simulink model "Switching_02"  (R2022b)
settings: Solver=ode4  StartTime=0.0  StopTime=50  FixedStep=1e-3  MaxStep=1e-3  RelTol=1e-3
undefined symbols (not defined in the file or in its folder): p1, p2, p3, PR_kv, PR_kw, SF_b, SF_xi1, v_sat, w_sat, x_d, y_d
libraries: simulink x18, dspsigops x6
settings Model: Creator=david  LastModifiedBy=david

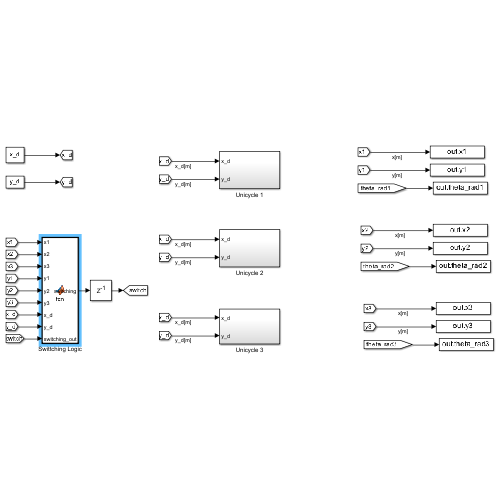
[thumbnail: Simulink's stored preview of the top-level diagram]
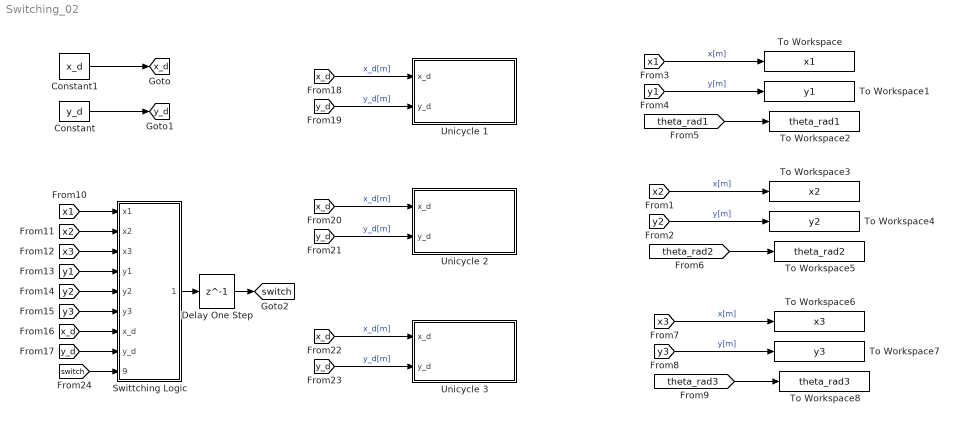
== system Switching_02 ==
  Constant : Constant  Value=y_d
  Constant1 : Constant  Value=x_d
  Delay One Step : Delay  DelayLength=1
  Swittching Logic : MATLAB Function  TreatAsAtomicUnit=on
  To Workspace : ToWorkspace  VariableName=x1  SaveFormat=Structure With Time  SampleTime=-1
  To Workspace1 : ToWorkspace  VariableName=y1  SaveFormat=Structure With Time  SampleTime=-1
  To Workspace2 : ToWorkspace  VariableName=theta_rad1  SaveFormat=Structure With Time  SampleTime=-1
  To Workspace3 : ToWorkspace  VariableName=x2  SaveFormat=Structure With Time  SampleTime=-1
  To Workspace4 : ToWorkspace  VariableName=y2  SaveFormat=Structure With Time  SampleTime=-1
  To Workspace5 : ToWorkspace  VariableName=theta_rad2  SaveFormat=Structure With Time  SampleTime=-1
  To Workspace6 : ToWorkspace  VariableName=x3  SaveFormat=Structure With Time  SampleTime=-1
  To Workspace7 : ToWorkspace  VariableName=y3  SaveFormat=Structure With Time  SampleTime=-1
  To Workspace8 : ToWorkspace  VariableName=theta_rad3  SaveFormat=Structure With Time  SampleTime=-1
  Unicycle 1 : Subsystem
  Unicycle 2 : Subsystem
  Unicycle 3 : Subsystem
  tag scope: switch=global, x_d=global, y_d=global
  wires:
  [x1] -> To Workspace/1  "x[m]"
  [y1] -> To Workspace1/1  "y[m]"
  [theta_rad1] -> To Workspace2/1
  [x2] -> To Workspace3/1  "x[m]"
  [y2] -> To Workspace4/1  "y[m]"
  [theta_rad2] -> To Workspace5/1
  [theta_rad3] -> To Workspace8/1
  [y3] -> To Workspace7/1  "y[m]"
  [x3] -> To Workspace6/1  "x[m]"
  Constant1/1 -> [x_d]
  Constant/1 -> [y_d]
  [x1] -> Swittching Logic/1(x1)
  [x2] -> Swittching Logic/2(x2)
  [x3] -> Swittching Logic/3(x3)
  [y1] -> Swittching Logic/4(y1)
  [y2] -> Swittching Logic/5(y2)
  [y3] -> Swittching Logic/6(y3)
  [x_d] -> Unicycle 1/1(x_d)  "x_d[m]"
  [y_d] -> Unicycle 1/2(y_d)  "y_d[m]"
  [y_d] -> Unicycle 2/2(y_d)  "y_d[m]"
  [x_d] -> Unicycle 2/1(x_d)  "x_d[m]"
  [y_d] -> Unicycle 3/2(y_d)  "y_d[m]"
  [x_d] -> Unicycle 3/1(x_d)  "x_d[m]"
  Swittching Logic/1(switching) -> Delay One Step/1
  [switch] -> Swittching Logic/9(switching_out)
  [y_d] -> Swittching Logic/8(y_d)
  [x_d] -> Swittching Logic/7(x_d)
  Delay One Step/1 -> [switch]

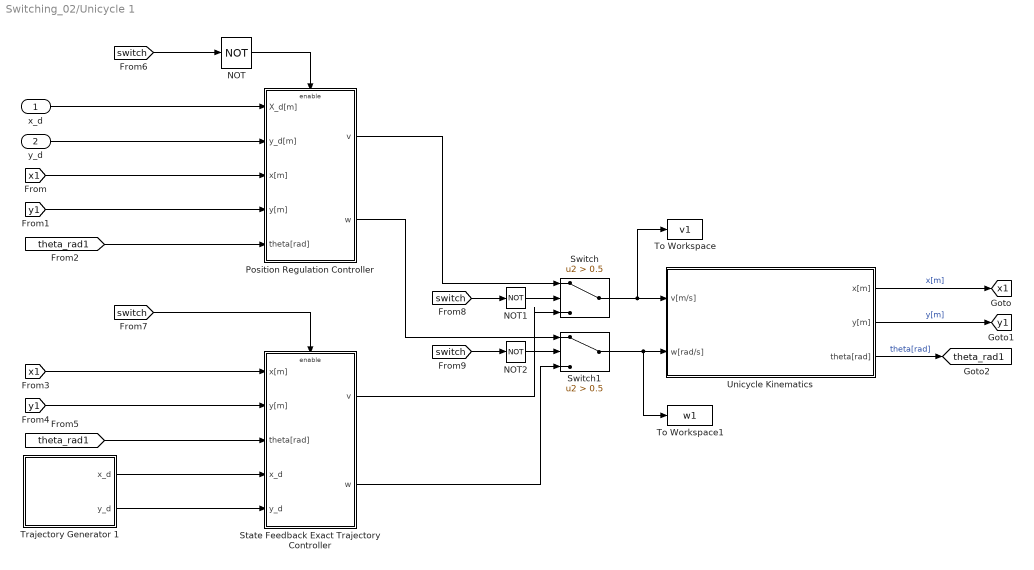
== system Switching_02/Unicycle 1 ==
  x_d : Inport
  y_d : Inport  Port=2
  NOT : Logic  Operator=NOT  IconShape=distinctive  AllPortsSameDT=off  OutDataTypeStr=boolean
  NOT1 : Logic  Operator=NOT  IconShape=distinctive  AllPortsSameDT=off  OutDataTypeStr=boolean
  NOT2 : Logic  Operator=NOT  IconShape=distinctive  AllPortsSameDT=off  OutDataTypeStr=boolean
  Position Regulation Controller : Subsystem
  State Feedback Exact Trajectory Controller : Subsystem
  Switch : Switch  Criteria=u2 > Threshold  Threshold=0.5  SaturateOnIntegerOverflow=off  InputSameDT=off
  Switch1 : Switch  Criteria=u2 > Threshold  Threshold=0.5  SaturateOnIntegerOverflow=off  InputSameDT=off
  To Workspace : ToWorkspace  VariableName=v1  SaveFormat=Structure With Time  SampleTime=-1
  To Workspace1 : ToWorkspace  VariableName=w1  SaveFormat=Structure With Time  SampleTime=-1
  "Trajectory Generator 1 " : Subsystem
  Unicycle Kinematics : Subsystem
  tag scope: theta_rad1=global, x1=global, y1=global
  wires:
  Unicycle Kinematics/3(theta[rad]) -> [theta_rad1]  "theta[rad]"
  [y1] -> Position Regulation Controller/4(y[m])
  [theta_rad1] -> Position Regulation Controller/5(theta[rad])
  Unicycle Kinematics/2(y[m]) -> [y1]  "y[m]"
  [x1] -> Position Regulation Controller/3(x[m])
  Unicycle Kinematics/1(x[m]) -> [x1]  "x[m]"
  x_d/1 -> Position Regulation Controller/1(X_d[m])
  y_d/1 -> Position Regulation Controller/2(y_d[m])
  [theta_rad1] -> State Feedback Exact Trajectory Controller/3(theta[rad])
  [x1] -> State Feedback Exact Trajectory Controller/1(x[m])
  [y1] -> State Feedback Exact Trajectory Controller/2(y[m])
  "Trajectory Generator 1 "/1(x_d) -> State Feedback Exact Trajectory Controller/4(x_d)
  "Trajectory Generator 1 "/2(y_d) -> State Feedback Exact Trajectory Controller/5(y_d)
  NOT/1 -> Position Regulation Controller/Enable
  [switch] -> NOT/1
  [switch] -> State Feedback Exact Trajectory Controller/Enable
  Position Regulation Controller/2(w) -> Switch1/1
  Position Regulation Controller/1(v) -> Switch/1
  State Feedback Exact Trajectory Controller/2(w) -> Switch1/3
  [switch] -> NOT2/1
  State Feedback Exact Trajectory Controller/1(v) -> Switch/3
  [switch] -> NOT1/1
  NOT1/1 -> Switch/2
  NOT2/1 -> Switch1/2
  Switch/1 -> Unicycle Kinematics/1(v[m/s]), To Workspace/1
  Switch1/1 -> Unicycle Kinematics/2(w[rad/s]), To Workspace1/1

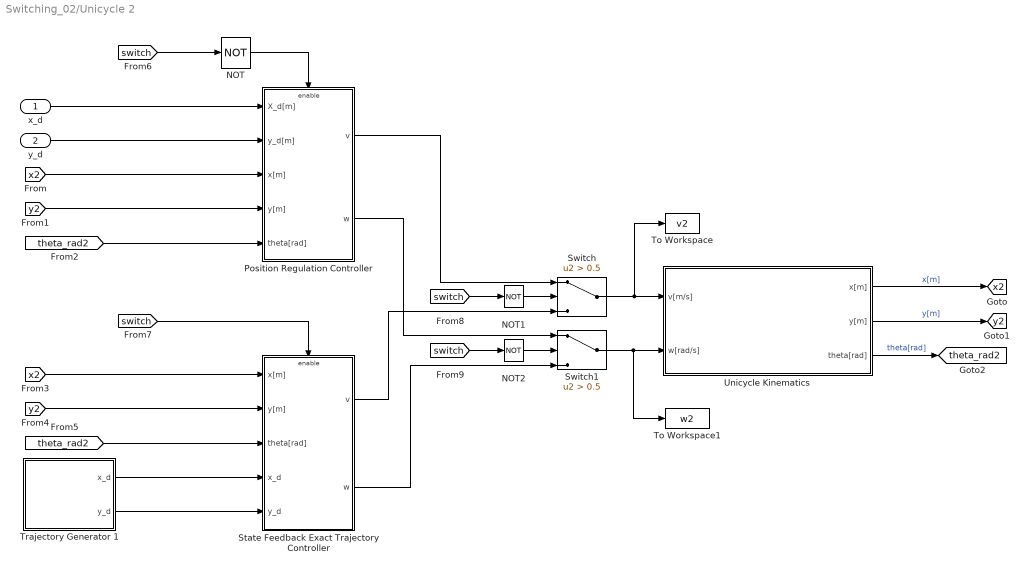
== system Switching_02/Unicycle 2 ==
  x_d : Inport
  y_d : Inport  Port=2
  NOT : Logic  Operator=NOT  IconShape=distinctive  AllPortsSameDT=off  OutDataTypeStr=boolean
  NOT1 : Logic  Operator=NOT  IconShape=distinctive  AllPortsSameDT=off  OutDataTypeStr=boolean
  NOT2 : Logic  Operator=NOT  IconShape=distinctive  AllPortsSameDT=off  OutDataTypeStr=boolean
  Position Regulation Controller : Subsystem
  State Feedback Exact Trajectory Controller : Subsystem
  Switch : Switch  Criteria=u2 > Threshold  Threshold=0.5  SaturateOnIntegerOverflow=off  InputSameDT=off
  Switch1 : Switch  Criteria=u2 > Threshold  Threshold=0.5  SaturateOnIntegerOverflow=off  InputSameDT=off
  To Workspace : ToWorkspace  VariableName=v2  SaveFormat=Structure With Time  SampleTime=-1
  To Workspace1 : ToWorkspace  VariableName=w2  SaveFormat=Structure With Time  SampleTime=-1
  "Trajectory Generator 1 " : Subsystem
  Unicycle Kinematics : Subsystem
  tag scope: theta_rad2=global, x2=global, y2=global
  wires:
  Unicycle Kinematics/3(theta[rad]) -> [theta_rad2]  "theta[rad]"
  [y2] -> Position Regulation Controller/4(y[m])
  [theta_rad2] -> Position Regulation Controller/5(theta[rad])
  Unicycle Kinematics/2(y[m]) -> [y2]  "y[m]"
  [x2] -> Position Regulation Controller/3(x[m])
  Unicycle Kinematics/1(x[m]) -> [x2]  "x[m]"
  x_d/1 -> Position Regulation Controller/1(X_d[m])
  y_d/1 -> Position Regulation Controller/2(y_d[m])
  NOT/1 -> Position Regulation Controller/Enable
  [switch] -> NOT/1
  [switch] -> State Feedback Exact Trajectory Controller/Enable
  Position Regulation Controller/2(w) -> Switch1/1
  Position Regulation Controller/1(v) -> Switch/1
  State Feedback Exact Trajectory Controller/2(w) -> Switch1/3
  [switch] -> NOT2/1
  Switch/1 -> To Workspace/1, Unicycle Kinematics/1(v[m/s])
  Switch1/1 -> To Workspace1/1, Unicycle Kinematics/2(w[rad/s])
  [switch] -> NOT1/1
  NOT1/1 -> Switch/2
  NOT2/1 -> Switch1/2
  State Feedback Exact Trajectory Controller/1(v) -> Switch/3
  [theta_rad2] -> State Feedback Exact Trajectory Controller/3(theta[rad])
  [x2] -> State Feedback Exact Trajectory Controller/1(x[m])
  [y2] -> State Feedback Exact Trajectory Controller/2(y[m])
  "Trajectory Generator 1 "/1(x_d) -> State Feedback Exact Trajectory Controller/4(x_d)
  "Trajectory Generator 1 "/2(y_d) -> State Feedback Exact Trajectory Controller/5(y_d)

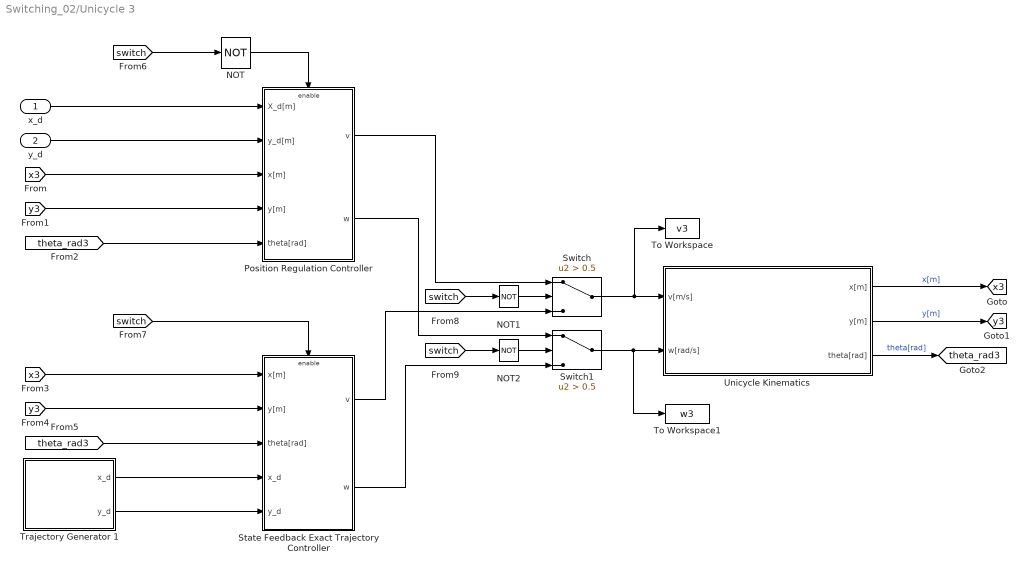
== system Switching_02/Unicycle 3 ==
  x_d : Inport
  y_d : Inport  Port=2
  NOT : Logic  Operator=NOT  IconShape=distinctive  AllPortsSameDT=off  OutDataTypeStr=boolean
  NOT1 : Logic  Operator=NOT  IconShape=distinctive  AllPortsSameDT=off  OutDataTypeStr=boolean
  NOT2 : Logic  Operator=NOT  IconShape=distinctive  AllPortsSameDT=off  OutDataTypeStr=boolean
  Position Regulation Controller : Subsystem
  State Feedback Exact Trajectory Controller : Subsystem
  Switch : Switch  Criteria=u2 > Threshold  Threshold=0.5  SaturateOnIntegerOverflow=off  InputSameDT=off
  Switch1 : Switch  Criteria=u2 > Threshold  Threshold=0.5  SaturateOnIntegerOverflow=off  InputSameDT=off
  To Workspace : ToWorkspace  VariableName=v3  SaveFormat=Structure With Time  SampleTime=-1
  To Workspace1 : ToWorkspace  VariableName=w3  SaveFormat=Structure With Time  SampleTime=-1
  "Trajectory Generator 1 " : Subsystem
  Unicycle Kinematics : Subsystem
  tag scope: theta_rad3=global, x3=global, y3=global
  wires:
  Unicycle Kinematics/3(theta[rad]) -> [theta_rad3]  "theta[rad]"
  [y3] -> Position Regulation Controller/4(y[m])
  [theta_rad3] -> Position Regulation Controller/5(theta[rad])
  Unicycle Kinematics/2(y[m]) -> [y3]  "y[m]"
  [x3] -> Position Regulation Controller/3(x[m])
  Unicycle Kinematics/1(x[m]) -> [x3]  "x[m]"
  x_d/1 -> Position Regulation Controller/1(X_d[m])
  y_d/1 -> Position Regulation Controller/2(y_d[m])
  NOT/1 -> Position Regulation Controller/Enable
  [switch] -> NOT/1
  [switch] -> State Feedback Exact Trajectory Controller/Enable
  Position Regulation Controller/1(v) -> Switch/1
  [switch] -> NOT1/1
  [switch] -> NOT2/1
  Position Regulation Controller/2(w) -> Switch1/1
  NOT1/1 -> Switch/2
  NOT2/1 -> Switch1/2
  [theta_rad3] -> State Feedback Exact Trajectory Controller/3(theta[rad])
  [x3] -> State Feedback Exact Trajectory Controller/1(x[m])
  [y3] -> State Feedback Exact Trajectory Controller/2(y[m])
  "Trajectory Generator 1 "/1(x_d) -> State Feedback Exact Trajectory Controller/4(x_d)
  "Trajectory Generator 1 "/2(y_d) -> State Feedback Exact Trajectory Controller/5(y_d)
  State Feedback Exact Trajectory Controller/1(v) -> Switch/3
  State Feedback Exact Trajectory Controller/2(w) -> Switch1/3
  Switch/1 -> Unicycle Kinematics/1(v[m/s]), To Workspace/1
  Switch1/1 -> To Workspace1/1, Unicycle Kinematics/2(w[rad/s])

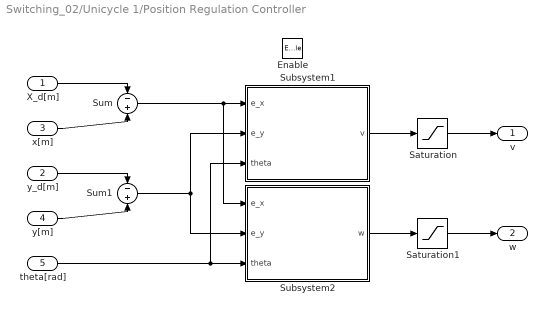
== system Switching_02/Unicycle 1/Position Regulation Controller ==
  X_d[m] : Inport
  y_d[m] : Inport  Port=2
  x[m] : Inport  Port=3
  y[m] : Inport  Port=4
  theta[rad] : Inport  Port=5
  Enable : EnablePort
  Saturation : Saturate  UpperLimit=v_sat  LowerLimit=-v_sat
  Saturation1 : Saturate  UpperLimit=w_sat  LowerLimit=-w_sat
  Subsystem1 : Subsystem
  Subsystem2 : Subsystem
  Sum : Sum  Inputs=-+
  Sum1 : Sum  Inputs=-+
  v : Outport
  w : Outport  Port=2
  wires:
  X_d[m]/1 -> Sum/1
  x[m]/1 -> Sum/2
  y_d[m]/1 -> Sum1/1
  y[m]/1 -> Sum1/2
  theta[rad]/1 -> Subsystem2/3(theta), Subsystem1/3(theta)
  Sum/1 -> Subsystem2/1(e_x), Subsystem1/1(e_x)
  Sum1/1 -> Subsystem1/2(e_y), Subsystem2/2(e_y)
  Subsystem2/1(w) -> Saturation1/1
  Subsystem1/1(v) -> Saturation/1
  Saturation/1 -> v/1
  Saturation1/1 -> w/1

== system Switching_02/Unicycle 1/State Feedback Exact Trajectory Controller ==
  x[m] : Inport
  y[m] : Inport  Port=2
  theta[rad] : Inport  Port=3
  x_d : Inport  Port=4
  y_d : Inport  Port=5
  Enable : EnablePort
  Controller : Subsystem
  Differential Flatness : Subsystem
  v : Outport
  w : Outport  Port=2
  wires:
  Controller/2(w) -> w/1
  Controller/1(v) -> v/1
  Differential Flatness/3(w_d) -> Controller/3(w_d)
  Differential Flatness/1(q_d) -> Controller/1(q_d)
  Differential Flatness/2(v_d) -> Controller/2(v_d)
  y_d/1 -> Differential Flatness/2(y_d)
  x_d/1 -> Differential Flatness/1(x_d)
  x[m]/1 -> Controller/4(x)
  y[m]/1 -> Controller/5(y)
  theta[rad]/1 -> Controller/6(theta)

== system Switching_02/Unicycle 1/Trajectory Generator 1  ==
  Repeating Sequence : simulink/Sources/Repeating Sequence  rep_seq_t=time  rep_seq_y=y_d1
  Repeating Sequence1 : simulink/Sources/Repeating Sequence  rep_seq_t=time  rep_seq_y=x_d1
  To Workspace2 : ToWorkspace  VariableName=y_d1  SaveFormat=Structure With Time  SampleTime=-1
  To Workspace3 : ToWorkspace  VariableName=x_d1  SaveFormat=Structure With Time  SampleTime=-1
  x_d : Outport
  y_d : Outport  Port=2
  wires:
  Repeating Sequence1/1 -> x_d/1, To Workspace3/1
  Repeating Sequence/1 -> To Workspace2/1, y_d/1

== system Switching_02/Unicycle 1/Unicycle Kinematics ==
  v[m/s] : Inport
  w[rad/s] : Inport  Port=2
  Cos : Trigonometry  Operator=cos
  Cos1 : Trigonometry
  Integrator : Integrator  InitialCondition=p1(1)
  Integrator1 : Integrator  InitialCondition=p1(2)
  Integrator2 : Integrator  InitialCondition=p1(3)
  Product : Product
  Product1 : Product
  x[m] : Outport
  y[m] : Outport  Port=2
  theta[rad] : Outport  Port=3
  wires:
  Integrator/1 -> x[m]/1  "x"
  Integrator1/1 -> y[m]/1  "y"
  w[rad/s]/1 -> Integrator2/1  "theta_dot"
  Integrator2/1 -> Cos/1, Cos1/1, theta[rad]/1  "theta[rad]"
  Product/1 -> Integrator/1  "x_dot"
  Cos1/1 -> Product1/2
  Cos/1 -> Product/1
  v[m/s]/1 -> Product1/1, Product/2
  Product1/1 -> Integrator1/1  "y_dot"

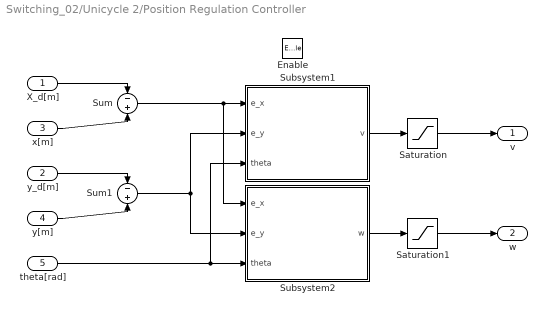
== system Switching_02/Unicycle 2/Position Regulation Controller ==
  X_d[m] : Inport
  y_d[m] : Inport  Port=2
  x[m] : Inport  Port=3
  y[m] : Inport  Port=4
  theta[rad] : Inport  Port=5
  Enable : EnablePort
  Saturation : Saturate  UpperLimit=v_sat  LowerLimit=-v_sat
  Saturation1 : Saturate  UpperLimit=w_sat  LowerLimit=-w_sat
  Subsystem1 : Subsystem
  Subsystem2 : Subsystem
  Sum : Sum  Inputs=-+
  Sum1 : Sum  Inputs=-+
  v : Outport
  w : Outport  Port=2
  wires:
  X_d[m]/1 -> Sum/1
  x[m]/1 -> Sum/2
  y_d[m]/1 -> Sum1/1
  y[m]/1 -> Sum1/2
  theta[rad]/1 -> Subsystem2/3(theta), Subsystem1/3(theta)
  Sum/1 -> Subsystem2/1(e_x), Subsystem1/1(e_x)
  Sum1/1 -> Subsystem1/2(e_y), Subsystem2/2(e_y)
  Subsystem2/1(w) -> Saturation1/1
  Subsystem1/1(v) -> Saturation/1
  Saturation/1 -> v/1
  Saturation1/1 -> w/1

== system Switching_02/Unicycle 2/State Feedback Exact Trajectory Controller ==
  x[m] : Inport
  y[m] : Inport  Port=2
  theta[rad] : Inport  Port=3
  x_d : Inport  Port=4
  y_d : Inport  Port=5
  Enable : EnablePort
  Controller : Subsystem
  Differential Flatness : Subsystem
  v : Outport
  w : Outport  Port=2
  wires:
  Controller/2(w) -> w/1
  Controller/1(v) -> v/1
  Differential Flatness/3(w_d) -> Controller/3(w_d)
  Differential Flatness/1(q_d) -> Controller/1(q_d)
  Differential Flatness/2(v_d) -> Controller/2(v_d)
  y_d/1 -> Differential Flatness/2(y_d)
  x_d/1 -> Differential Flatness/1(x_d)
  x[m]/1 -> Controller/4(x)
  y[m]/1 -> Controller/5(y)
  theta[rad]/1 -> Controller/6(theta)

== system Switching_02/Unicycle 2/Trajectory Generator 1  ==
  Repeating Sequence : simulink/Sources/Repeating Sequence  rep_seq_t=time  rep_seq_y=y_d2
  Repeating Sequence1 : simulink/Sources/Repeating Sequence  rep_seq_t=time  rep_seq_y=x_d2
  To Workspace2 : ToWorkspace  VariableName=y_d2  SaveFormat=Structure With Time  SampleTime=-1
  To Workspace3 : ToWorkspace  VariableName=x_d2  SaveFormat=Structure With Time  SampleTime=-1
  x_d : Outport
  y_d : Outport  Port=2
  wires:
  Repeating Sequence1/1 -> x_d/1, To Workspace3/1
  Repeating Sequence/1 -> To Workspace2/1, y_d/1

== system Switching_02/Unicycle 2/Unicycle Kinematics ==
  v[m/s] : Inport
  w[rad/s] : Inport  Port=2
  Cos : Trigonometry  Operator=cos
  Cos1 : Trigonometry
  Integrator : Integrator  InitialCondition=p2(1)
  Integrator1 : Integrator  InitialCondition=p2(2)
  Integrator2 : Integrator  InitialCondition=p2(3)
  Product : Product
  Product1 : Product
  x[m] : Outport
  y[m] : Outport  Port=2
  theta[rad] : Outport  Port=3
  wires:
  Integrator/1 -> x[m]/1  "x"
  Integrator1/1 -> y[m]/1  "y"
  w[rad/s]/1 -> Integrator2/1  "theta_dot"
  Integrator2/1 -> Cos/1, Cos1/1, theta[rad]/1  "theta[rad]"
  Product/1 -> Integrator/1  "x_dot"
  Cos1/1 -> Product1/2
  Cos/1 -> Product/1
  v[m/s]/1 -> Product1/1, Product/2
  Product1/1 -> Integrator1/1  "y_dot"

== system Switching_02/Unicycle 3/Position Regulation Controller ==
  X_d[m] : Inport
  y_d[m] : Inport  Port=2
  x[m] : Inport  Port=3
  y[m] : Inport  Port=4
  theta[rad] : Inport  Port=5
  Enable : EnablePort
  Saturation : Saturate  UpperLimit=v_sat  LowerLimit=-v_sat
  Saturation1 : Saturate  UpperLimit=w_sat  LowerLimit=-w_sat
  Subsystem1 : Subsystem
  Subsystem2 : Subsystem
  Sum : Sum  Inputs=-+
  Sum1 : Sum  Inputs=-+
  v : Outport
  w : Outport  Port=2
  wires:
  X_d[m]/1 -> Sum/1
  x[m]/1 -> Sum/2
  y_d[m]/1 -> Sum1/1
  y[m]/1 -> Sum1/2
  theta[rad]/1 -> Subsystem2/3(theta), Subsystem1/3(theta)
  Sum/1 -> Subsystem2/1(e_x), Subsystem1/1(e_x)
  Sum1/1 -> Subsystem1/2(e_y), Subsystem2/2(e_y)
  Subsystem2/1(w) -> Saturation1/1
  Subsystem1/1(v) -> Saturation/1
  Saturation/1 -> v/1
  Saturation1/1 -> w/1

== system Switching_02/Unicycle 3/State Feedback Exact Trajectory Controller ==
  x[m] : Inport
  y[m] : Inport  Port=2
  theta[rad] : Inport  Port=3
  x_d : Inport  Port=4
  y_d : Inport  Port=5
  Enable : EnablePort
  Controller : Subsystem
  Differential Flatness : Subsystem
  v : Outport
  w : Outport  Port=2
  wires:
  Controller/2(w) -> w/1
  Controller/1(v) -> v/1
  Differential Flatness/3(w_d) -> Controller/3(w_d)
  Differential Flatness/1(q_d) -> Controller/1(q_d)
  Differential Flatness/2(v_d) -> Controller/2(v_d)
  y_d/1 -> Differential Flatness/2(y_d)
  x_d/1 -> Differential Flatness/1(x_d)
  x[m]/1 -> Controller/4(x)
  y[m]/1 -> Controller/5(y)
  theta[rad]/1 -> Controller/6(theta)

== system Switching_02/Unicycle 3/Trajectory Generator 1  ==
  Repeating Sequence : simulink/Sources/Repeating Sequence  rep_seq_t=time  rep_seq_y=y_d3
  Repeating Sequence1 : simulink/Sources/Repeating Sequence  rep_seq_t=time  rep_seq_y=x_d3
  To Workspace2 : ToWorkspace  VariableName=y_d3  SaveFormat=Structure With Time  SampleTime=-1
  To Workspace3 : ToWorkspace  VariableName=x_d3  SaveFormat=Structure With Time  SampleTime=-1
  x_d : Outport
  y_d : Outport  Port=2
  wires:
  Repeating Sequence1/1 -> x_d/1, To Workspace3/1
  Repeating Sequence/1 -> y_d/1, To Workspace2/1

== system Switching_02/Unicycle 3/Unicycle Kinematics ==
  v[m/s] : Inport
  w[rad/s] : Inport  Port=2
  Cos : Trigonometry  Operator=cos
  Cos1 : Trigonometry
  Integrator : Integrator  InitialCondition=p3(1)
  Integrator1 : Integrator  InitialCondition=p3(2)
  Integrator2 : Integrator  InitialCondition=p3(3)
  Product : Product
  Product1 : Product
  x[m] : Outport
  y[m] : Outport  Port=2
  theta[rad] : Outport  Port=3
  wires:
  Integrator/1 -> x[m]/1  "x"
  Integrator1/1 -> y[m]/1  "y"
  w[rad/s]/1 -> Integrator2/1  "theta_dot"
  Integrator2/1 -> Cos/1, Cos1/1, theta[rad]/1  "theta[rad]"
  Product/1 -> Integrator/1  "x_dot"
  Cos1/1 -> Product1/2
  Cos/1 -> Product/1
  v[m/s]/1 -> Product1/1, Product/2
  Product1/1 -> Integrator1/1  "y_dot"

== system Switching_02/Unicycle 1/Position Regulation Controller/Subsystem1 ==
  e_x : Inport
  e_y : Inport  Port=2
  theta : Inport  Port=3
  Gain : Gain  Gain=PR_kv
  Product : Product
  Product1 : Product
  Sin : Trigonometry
  Sin1 : Trigonometry  Operator=cos
  Sum : Sum  Inputs=--
  v : Outport
  wires:
  e_y/1 -> Product/2
  theta/1 -> Sin/1, Sin1/1
  Sum/1 -> Gain/1
  Gain/1 -> v/1
  Sin/1 -> Product/1
  Product/1 -> Sum/2
  e_x/1 -> Product1/1
  Sin1/1 -> Product1/2
  Product1/1 -> Sum/1

== system Switching_02/Unicycle 1/Position Regulation Controller/Subsystem2 ==
  e_x : Inport
  e_y : Inport  Port=2
  theta : Inport  Port=3
  Atan2 : Trigonometry  Operator=atan2  ApproximationMethod=Lookup  NumberOfDataPoints=2
  Constant : Constant  Value=pi
  Gain : Gain  Gain=PR_kw
  Sum : Sum  Inputs=+-+
  Unwrap : dspsigops/Unwrap  tol=pi  InputProcessing=Columns as channels (frame based)  running=off
  w : Outport
  wires:
  e_x/1 -> Atan2/2
  e_y/1 -> Atan2/1
  theta/1 -> Sum/2
  Sum/1 -> Gain/1
  Atan2/1 -> Unwrap/1
  Constant/1 -> Sum/3
  Gain/1 -> w/1
  Unwrap/1 -> Sum/1

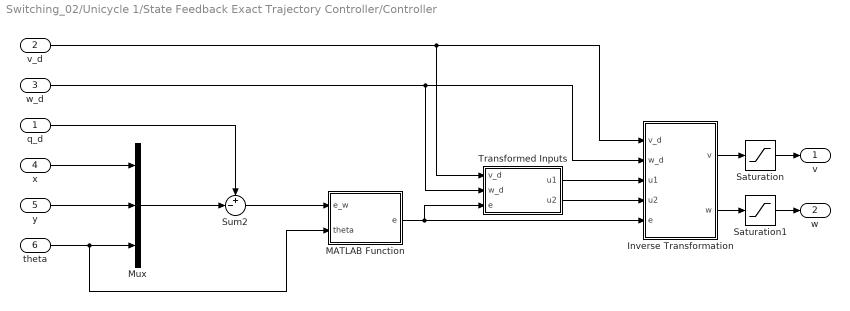
== system Switching_02/Unicycle 1/State Feedback Exact Trajectory Controller/Controller ==
  q_d : Inport
  v_d : Inport  Port=2
  w_d : Inport  Port=3
  x : Inport  Port=4
  y : Inport  Port=5
  theta : Inport  Port=6
  Inverse Transformation : MATLAB Function  TreatAsAtomicUnit=on
  MATLAB Function : MATLAB Function  TreatAsAtomicUnit=on
  Mux : Mux  Inputs=3
  Saturation : Saturate  UpperLimit=v_sat  LowerLimit=-v_sat
  Saturation1 : Saturate  UpperLimit=w_sat  LowerLimit=-w_sat
  Sum2 : Sum  Inputs=+-|
  Transformed Inputs : MATLAB Function  TreatAsAtomicUnit=on
  v : Outport
  w : Outport  Port=2
  wires:
  q_d/1 -> Sum2/1
  MATLAB Function/1(e) -> Inverse Transformation/5(e), Transformed Inputs/3(e)
  Transformed Inputs/1(u1) -> Inverse Transformation/3(u1)
  Transformed Inputs/2(u2) -> Inverse Transformation/4(u2)
  Inverse Transformation/1(v) -> Saturation/1
  Inverse Transformation/2(w) -> Saturation1/1
  x/1 -> Mux/1
  y/1 -> Mux/2
  theta/1 -> Mux/3, MATLAB Function/2(theta)
  Mux/1 -> Sum2/2
  Sum2/1 -> MATLAB Function/1(e_w)
  w_d/1 -> Inverse Transformation/2(w_d), Transformed Inputs/2(w_d)
  v_d/1 -> Transformed Inputs/1(v_d), Inverse Transformation/1(v_d)
  Saturation/1 -> v/1
  Saturation1/1 -> w/1

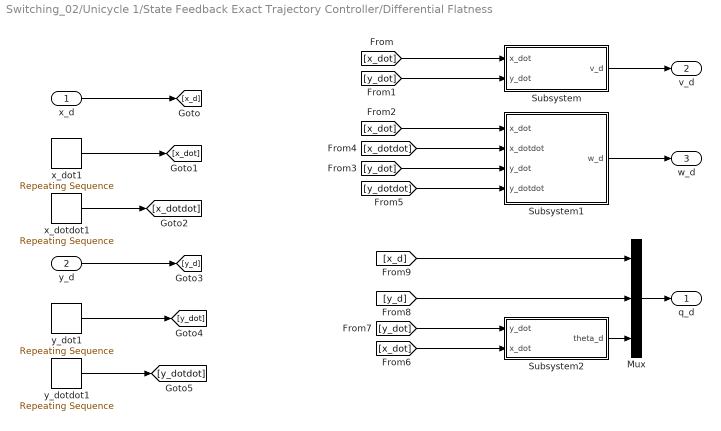
== system Switching_02/Unicycle 1/State Feedback Exact Trajectory Controller/Differential Flatness ==
  x_d : Inport
  y_d : Inport  Port=2
  Mux : Mux  Inputs=3
  Subsystem : Subsystem
  Subsystem1 : Subsystem
  Subsystem2 : Subsystem
  x_dot1 : simulink/Sources/Repeating Sequence  rep_seq_t=time  rep_seq_y=x_dot1
  x_dotdot1 : simulink/Sources/Repeating Sequence  rep_seq_t=time  rep_seq_y=x_dotdot1
  y_dot1 : simulink/Sources/Repeating Sequence  rep_seq_t=time  rep_seq_y=y_dot1
  y_dotdot1 : simulink/Sources/Repeating Sequence  rep_seq_t=time  rep_seq_y=y_dotdot1
  q_d : Outport
  v_d : Outport  Port=2
  w_d : Outport  Port=3
  wires:
  Subsystem/1(v_d) -> v_d/1
  [x_dot] -> Subsystem/1(x_dot)
  [y_dot] -> Subsystem/2(y_dot)
  [x_dot] -> Subsystem1/1(x_dot)
  [x_dotdot] -> Subsystem1/2(x_dotdot)
  Subsystem1/1(w_d) -> w_d/1
  [y_dot] -> Subsystem1/3(y_dot)
  [y_dotdot] -> Subsystem1/4(y_dotdot)
  Subsystem2/1(theta_d) -> Mux/3
  [y_d] -> Mux/2
  [x_d] -> Mux/1
  Mux/1 -> q_d/1
  [y_dot] -> Subsystem2/1(y_dot)
  [x_dot] -> Subsystem2/2(x_dot)
  y_d/1 -> [y_d]
  y_dotdot1/1 -> [y_dotdot]
  x_dot1/1 -> [x_dot]
  x_d/1 -> [x_d]
  y_dot1/1 -> [y_dot]
  x_dotdot1/1 -> [x_dotdot]

== system Switching_02/Unicycle 2/Position Regulation Controller/Subsystem1 ==
  e_x : Inport
  e_y : Inport  Port=2
  theta : Inport  Port=3
  Gain : Gain  Gain=PR_kv
  Product : Product
  Product1 : Product
  Sin : Trigonometry
  Sin1 : Trigonometry  Operator=cos
  Sum : Sum  Inputs=--
  v : Outport
  wires:
  e_y/1 -> Product/2
  theta/1 -> Sin/1, Sin1/1
  Sum/1 -> Gain/1
  Gain/1 -> v/1
  Sin/1 -> Product/1
  Product/1 -> Sum/2
  e_x/1 -> Product1/1
  Sin1/1 -> Product1/2
  Product1/1 -> Sum/1

== system Switching_02/Unicycle 2/Position Regulation Controller/Subsystem2 ==
  e_x : Inport
  e_y : Inport  Port=2
  theta : Inport  Port=3
  Atan2 : Trigonometry  Operator=atan2  ApproximationMethod=Lookup  NumberOfDataPoints=2
  Constant : Constant  Value=pi
  Gain : Gain  Gain=PR_kw
  Sum : Sum  Inputs=+-+
  Unwrap : dspsigops/Unwrap  tol=pi  InputProcessing=Columns as channels (frame based)  running=off
  w : Outport
  wires:
  e_x/1 -> Atan2/2
  e_y/1 -> Atan2/1
  theta/1 -> Sum/2
  Sum/1 -> Gain/1
  Atan2/1 -> Unwrap/1
  Constant/1 -> Sum/3
  Gain/1 -> w/1
  Unwrap/1 -> Sum/1

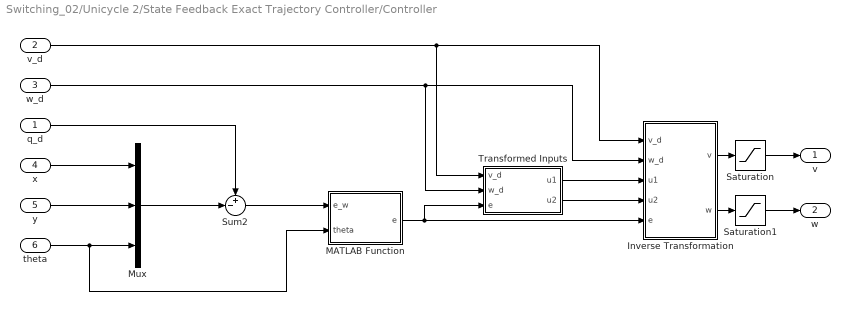
== system Switching_02/Unicycle 2/State Feedback Exact Trajectory Controller/Controller ==
  q_d : Inport
  v_d : Inport  Port=2
  w_d : Inport  Port=3
  x : Inport  Port=4
  y : Inport  Port=5
  theta : Inport  Port=6
  Inverse Transformation : MATLAB Function  TreatAsAtomicUnit=on
  MATLAB Function : MATLAB Function  TreatAsAtomicUnit=on
  Mux : Mux  Inputs=3
  Saturation : Saturate  UpperLimit=v_sat  LowerLimit=-v_sat
  Saturation1 : Saturate  UpperLimit=w_sat  LowerLimit=-w_sat
  Sum2 : Sum  Inputs=+-|
  Transformed Inputs : MATLAB Function  TreatAsAtomicUnit=on
  v : Outport
  w : Outport  Port=2
  wires:
  q_d/1 -> Sum2/1
  MATLAB Function/1(e) -> Inverse Transformation/5(e), Transformed Inputs/3(e)
  Transformed Inputs/1(u1) -> Inverse Transformation/3(u1)
  Transformed Inputs/2(u2) -> Inverse Transformation/4(u2)
  Inverse Transformation/1(v) -> Saturation/1
  Inverse Transformation/2(w) -> Saturation1/1
  x/1 -> Mux/1
  y/1 -> Mux/2
  theta/1 -> Mux/3, MATLAB Function/2(theta)
  Mux/1 -> Sum2/2
  Sum2/1 -> MATLAB Function/1(e_w)
  w_d/1 -> Inverse Transformation/2(w_d), Transformed Inputs/2(w_d)
  v_d/1 -> Transformed Inputs/1(v_d), Inverse Transformation/1(v_d)
  Saturation/1 -> v/1
  Saturation1/1 -> w/1

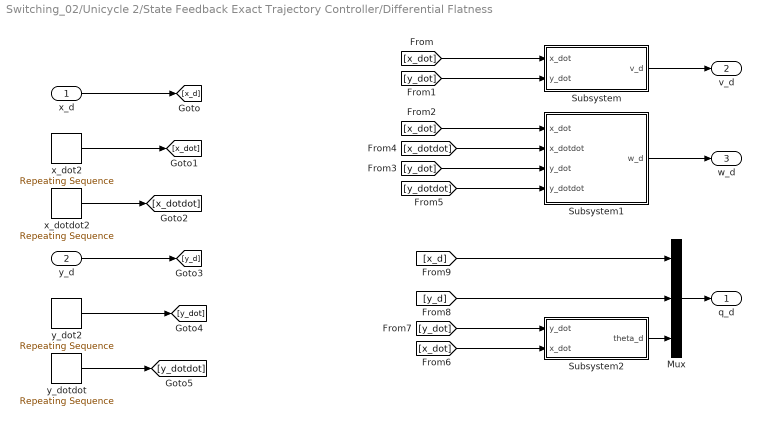
== system Switching_02/Unicycle 2/State Feedback Exact Trajectory Controller/Differential Flatness ==
  x_d : Inport
  y_d : Inport  Port=2
  Mux : Mux  Inputs=3
  Subsystem : Subsystem
  Subsystem1 : Subsystem
  Subsystem2 : Subsystem
  x_dot2 : simulink/Sources/Repeating Sequence  rep_seq_t=time  rep_seq_y=x_dot2
  x_dotdot2 : simulink/Sources/Repeating Sequence  rep_seq_t=time  rep_seq_y=x_dotdot2
  y_dot2 : simulink/Sources/Repeating Sequence  rep_seq_t=time  rep_seq_y=y_dot2
  y_dotdot : simulink/Sources/Repeating Sequence  rep_seq_t=time  rep_seq_y=y_dotdot2
  q_d : Outport
  v_d : Outport  Port=2
  w_d : Outport  Port=3
  wires:
  Subsystem/1(v_d) -> v_d/1
  [x_dot] -> Subsystem/1(x_dot)
  [y_dot] -> Subsystem/2(y_dot)
  [x_dot] -> Subsystem1/1(x_dot)
  [x_dotdot] -> Subsystem1/2(x_dotdot)
  Subsystem1/1(w_d) -> w_d/1
  [y_dot] -> Subsystem1/3(y_dot)
  [y_dotdot] -> Subsystem1/4(y_dotdot)
  Subsystem2/1(theta_d) -> Mux/3
  [y_d] -> Mux/2
  [x_d] -> Mux/1
  Mux/1 -> q_d/1
  [y_dot] -> Subsystem2/1(y_dot)
  [x_dot] -> Subsystem2/2(x_dot)
  y_d/1 -> [y_d]
  x_dotdot2/1 -> [x_dotdot]
  x_d/1 -> [x_d]
  x_dot2/1 -> [x_dot]
  y_dotdot/1 -> [y_dotdot]
  y_dot2/1 -> [y_dot]

== system Switching_02/Unicycle 3/Position Regulation Controller/Subsystem1 ==
  e_x : Inport
  e_y : Inport  Port=2
  theta : Inport  Port=3
  Gain : Gain  Gain=PR_kv
  Product : Product
  Product1 : Product
  Sin : Trigonometry
  Sin1 : Trigonometry  Operator=cos
  Sum : Sum  Inputs=--
  v : Outport
  wires:
  e_y/1 -> Product/2
  theta/1 -> Sin/1, Sin1/1
  Sum/1 -> Gain/1
  Gain/1 -> v/1
  Sin/1 -> Product/1
  Product/1 -> Sum/2
  e_x/1 -> Product1/1
  Sin1/1 -> Product1/2
  Product1/1 -> Sum/1

== system Switching_02/Unicycle 3/Position Regulation Controller/Subsystem2 ==
  e_x : Inport
  e_y : Inport  Port=2
  theta : Inport  Port=3
  Atan2 : Trigonometry  Operator=atan2  ApproximationMethod=Lookup  NumberOfDataPoints=2
  Constant : Constant  Value=pi
  Gain : Gain  Gain=PR_kw
  Sum : Sum  Inputs=+-+
  Unwrap : dspsigops/Unwrap  tol=pi  InputProcessing=Columns as channels (frame based)  running=off
  w : Outport
  wires:
  e_x/1 -> Atan2/2
  e_y/1 -> Atan2/1
  theta/1 -> Sum/2
  Sum/1 -> Gain/1
  Atan2/1 -> Unwrap/1
  Constant/1 -> Sum/3
  Gain/1 -> w/1
  Unwrap/1 -> Sum/1

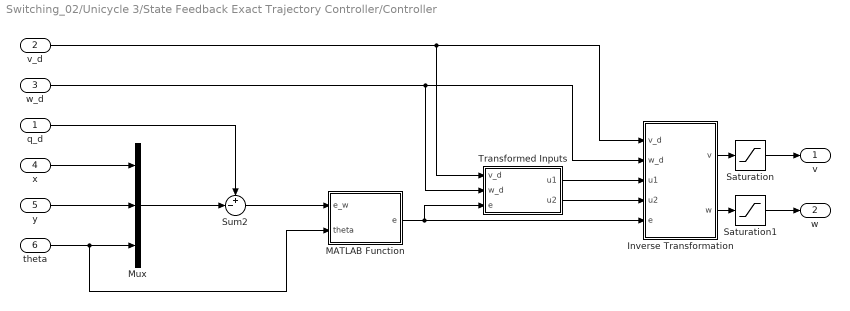
== system Switching_02/Unicycle 3/State Feedback Exact Trajectory Controller/Controller ==
  q_d : Inport
  v_d : Inport  Port=2
  w_d : Inport  Port=3
  x : Inport  Port=4
  y : Inport  Port=5
  theta : Inport  Port=6
  Inverse Transformation : MATLAB Function  TreatAsAtomicUnit=on
  MATLAB Function : MATLAB Function  TreatAsAtomicUnit=on
  Mux : Mux  Inputs=3
  Saturation : Saturate  UpperLimit=v_sat  LowerLimit=-v_sat
  Saturation1 : Saturate  UpperLimit=w_sat  LowerLimit=-w_sat
  Sum2 : Sum  Inputs=+-|
  Transformed Inputs : MATLAB Function  TreatAsAtomicUnit=on
  v : Outport
  w : Outport  Port=2
  wires:
  q_d/1 -> Sum2/1
  MATLAB Function/1(e) -> Inverse Transformation/5(e), Transformed Inputs/3(e)
  Transformed Inputs/1(u1) -> Inverse Transformation/3(u1)
  Transformed Inputs/2(u2) -> Inverse Transformation/4(u2)
  Inverse Transformation/1(v) -> Saturation/1
  Inverse Transformation/2(w) -> Saturation1/1
  x/1 -> Mux/1
  y/1 -> Mux/2
  theta/1 -> Mux/3, MATLAB Function/2(theta)
  Mux/1 -> Sum2/2
  Sum2/1 -> MATLAB Function/1(e_w)
  w_d/1 -> Inverse Transformation/2(w_d), Transformed Inputs/2(w_d)
  v_d/1 -> Transformed Inputs/1(v_d), Inverse Transformation/1(v_d)
  Saturation/1 -> v/1
  Saturation1/1 -> w/1

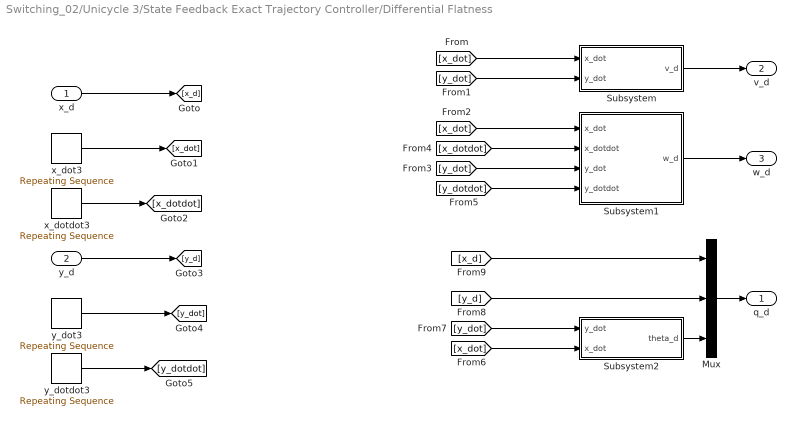
== system Switching_02/Unicycle 3/State Feedback Exact Trajectory Controller/Differential Flatness ==
  x_d : Inport
  y_d : Inport  Port=2
  Mux : Mux  Inputs=3
  Subsystem : Subsystem
  Subsystem1 : Subsystem
  Subsystem2 : Subsystem
  x_dot3 : simulink/Sources/Repeating Sequence  rep_seq_t=time  rep_seq_y=x_dot3
  x_dotdot3 : simulink/Sources/Repeating Sequence  rep_seq_t=time  rep_seq_y=x_dotdot3
  y_dot3 : simulink/Sources/Repeating Sequence  rep_seq_t=time  rep_seq_y=y_dot3
  y_dotdot3 : simulink/Sources/Repeating Sequence  rep_seq_t=time  rep_seq_y=y_dotdot3
  q_d : Outport
  v_d : Outport  Port=2
  w_d : Outport  Port=3
  wires:
  Subsystem/1(v_d) -> v_d/1
  [x_dot] -> Subsystem/1(x_dot)
  [y_dot] -> Subsystem/2(y_dot)
  [x_dot] -> Subsystem1/1(x_dot)
  [x_dotdot] -> Subsystem1/2(x_dotdot)
  Subsystem1/1(w_d) -> w_d/1
  [y_dot] -> Subsystem1/3(y_dot)
  [y_dotdot] -> Subsystem1/4(y_dotdot)
  Subsystem2/1(theta_d) -> Mux/3
  [y_d] -> Mux/2
  [x_d] -> Mux/1
  Mux/1 -> q_d/1
  [y_dot] -> Subsystem2/1(y_dot)
  [x_dot] -> Subsystem2/2(x_dot)
  y_dot3/1 -> [y_dot]
  y_dotdot3/1 -> [y_dotdot]
  x_d/1 -> [x_d]
  y_d/1 -> [y_d]
  x_dotdot3/1 -> [x_dotdot]
  x_dot3/1 -> [x_dot]

== system Switching_02/Unicycle 1/State Feedback Exact Trajectory Controller/Differential Flatness/Subsystem ==
  x_dot : Inport
  y_dot : Inport  Port=2
  Square : Math  Operator=square
  Square Root : Sqrt
  Square1 : Math  Operator=square
  Sum : Sum
  v_d : Outport
  wires:
  x_dot/1 -> Square/1
  y_dot/1 -> Square1/1
  Square/1 -> Sum/1
  Square1/1 -> Sum/2
  Square Root/1 -> v_d/1
  Sum/1 -> Square Root/1

== system Switching_02/Unicycle 1/State Feedback Exact Trajectory Controller/Differential Flatness/Subsystem1 ==
  x_dot : Inport
  x_dotdot : Inport  Port=2
  y_dot : Inport  Port=3
  y_dotdot : Inport  Port=4
  Divide : Product  Inputs=*/
  MATLAB Function : MATLAB Function  TreatAsAtomicUnit=on
  Product : Product
  Product1 : Product
  Square : Math  Operator=square
  Square1 : Math  Operator=square
  Sum : Sum  Inputs=+-
  Sum1 : Sum
  w_d : Outport
  wires:
  Product/1 -> Sum/1
  Product1/1 -> Sum/2
  Sum/1 -> Divide/1
  Divide/1 -> w_d/1
  x_dot/1 -> Square/1, Product/1
  y_dotdot/1 -> Product/2
  y_dot/1 -> Product1/2, Square1/1
  MATLAB Function/1(u) -> Divide/2
  Sum1/1 -> MATLAB Function/1("u ")
  Square/1 -> Sum1/1
  Square1/1 -> Sum1/2
  x_dotdot/1 -> Product1/1

== system Switching_02/Unicycle 1/State Feedback Exact Trajectory Controller/Differential Flatness/Subsystem2 ==
  y_dot : Inport
  x_dot : Inport  Port=2
  Atan2 : Trigonometry  Operator=atan2
  Unwrap : dspsigops/Unwrap  tol=pi  InputProcessing=Columns as channels (frame based)  running=off
  theta_d : Outport
  wires:
  Atan2/1 -> Unwrap/1
  y_dot/1 -> Atan2/1
  x_dot/1 -> Atan2/2
  Unwrap/1 -> theta_d/1

== system Switching_02/Unicycle 2/State Feedback Exact Trajectory Controller/Differential Flatness/Subsystem ==
  x_dot : Inport
  y_dot : Inport  Port=2
  Square : Math  Operator=square
  Square Root : Sqrt
  Square1 : Math  Operator=square
  Sum : Sum
  v_d : Outport
  wires:
  x_dot/1 -> Square/1
  y_dot/1 -> Square1/1
  Square/1 -> Sum/1
  Square1/1 -> Sum/2
  Square Root/1 -> v_d/1
  Sum/1 -> Square Root/1

== system Switching_02/Unicycle 2/State Feedback Exact Trajectory Controller/Differential Flatness/Subsystem1 ==
  x_dot : Inport
  x_dotdot : Inport  Port=2
  y_dot : Inport  Port=3
  y_dotdot : Inport  Port=4
  Divide : Product  Inputs=*/
  MATLAB Function : MATLAB Function  TreatAsAtomicUnit=on
  Product : Product
  Product1 : Product
  Square : Math  Operator=square
  Square1 : Math  Operator=square
  Sum : Sum  Inputs=+-
  Sum1 : Sum
  w_d : Outport
  wires:
  Product/1 -> Sum/1
  Product1/1 -> Sum/2
  Sum/1 -> Divide/1
  Divide/1 -> w_d/1
  x_dot/1 -> Square/1, Product/1
  y_dotdot/1 -> Product/2
  y_dot/1 -> Product1/2, Square1/1
  MATLAB Function/1(u) -> Divide/2
  Sum1/1 -> MATLAB Function/1("u ")
  Square/1 -> Sum1/1
  Square1/1 -> Sum1/2
  x_dotdot/1 -> Product1/1

== system Switching_02/Unicycle 2/State Feedback Exact Trajectory Controller/Differential Flatness/Subsystem2 ==
  y_dot : Inport
  x_dot : Inport  Port=2
  Atan2 : Trigonometry  Operator=atan2
  Unwrap : dspsigops/Unwrap  tol=pi  InputProcessing=Columns as channels (frame based)  running=off
  theta_d : Outport
  wires:
  Atan2/1 -> Unwrap/1
  y_dot/1 -> Atan2/1
  x_dot/1 -> Atan2/2
  Unwrap/1 -> theta_d/1

== system Switching_02/Unicycle 3/State Feedback Exact Trajectory Controller/Differential Flatness/Subsystem ==
  x_dot : Inport
  y_dot : Inport  Port=2
  Square : Math  Operator=square
  Square Root : Sqrt
  Square1 : Math  Operator=square
  Sum : Sum
  v_d : Outport
  wires:
  x_dot/1 -> Square/1
  y_dot/1 -> Square1/1
  Square/1 -> Sum/1
  Square1/1 -> Sum/2
  Square Root/1 -> v_d/1
  Sum/1 -> Square Root/1

== system Switching_02/Unicycle 3/State Feedback Exact Trajectory Controller/Differential Flatness/Subsystem1 ==
  x_dot : Inport
  x_dotdot : Inport  Port=2
  y_dot : Inport  Port=3
  y_dotdot : Inport  Port=4
  Divide : Product  Inputs=*/
  MATLAB Function : MATLAB Function  TreatAsAtomicUnit=on
  Product : Product
  Product1 : Product
  Square : Math  Operator=square
  Square1 : Math  Operator=square
  Sum : Sum  Inputs=+-
  Sum1 : Sum
  w_d : Outport
  wires:
  Product/1 -> Sum/1
  Product1/1 -> Sum/2
  Sum/1 -> Divide/1
  Divide/1 -> w_d/1
  x_dot/1 -> Square/1, Product/1
  y_dotdot/1 -> Product/2
  y_dot/1 -> Product1/2, Square1/1
  MATLAB Function/1(u) -> Divide/2
  Sum1/1 -> MATLAB Function/1("u ")
  Square/1 -> Sum1/1
  Square1/1 -> Sum1/2
  x_dotdot/1 -> Product1/1

== system Switching_02/Unicycle 3/State Feedback Exact Trajectory Controller/Differential Flatness/Subsystem2 ==
  y_dot : Inport
  x_dot : Inport  Port=2
  Atan2 : Trigonometry  Operator=atan2
  Unwrap : dspsigops/Unwrap  tol=pi  InputProcessing=Columns as channels (frame based)  running=off
  theta_d : Outport
  wires:
  Atan2/1 -> Unwrap/1
  y_dot/1 -> Atan2/1
  x_dot/1 -> Atan2/2
  Unwrap/1 -> theta_d/1

== matlab function Switching_02/Unicycle 1/State Feedback Exact Trajectory Controller/Differential Flatness/Subsystem1/MATLAB Function ==
  data: u input; u output
function u = fcn(u)

if abs(u)<1e-4
    if u>=0
        u=1e-4;
    else
        u=-1e-4;
    end
else
    u=u;
end

== matlab function Switching_02/Unicycle 2/State Feedback Exact Trajectory Controller/Controller/Transformed Inputs ==
  data: SF_b parameter; SF_xi1 parameter; v_d input; w_d input; e input; u1 output; u2 output
function [u1, u2] = fcn(SF_b, SF_xi1, v_d, w_d, e)

% calculatring values of K
k_1=2*SF_xi1*sqrt(SF_b*v_d+w_d^2);
k_2=SF_b;
k_3=k_1;

% calculating values of u
u1=-k_1*e(1);
u2=-k_2*(v_d*(sin(e(3))/e(3)))*e(2)-k_3*e(3);

== matlab function Switching_02/Unicycle 2/State Feedback Exact Trajectory Controller/Differential Flatness/Subsystem1/MATLAB Function ==
  data: u input; u output
function u = fcn(u)

if abs(u)<1e-4
    if u>=0
        u=1e-4;
    else
        u=-1e-4;
    end
else
    u=u;
end

== matlab function Switching_02/Unicycle 3/State Feedback Exact Trajectory Controller/Controller/MATLAB Function ==
  data: e_w input; e output; theta input
function e  = fcn(e_w, theta)

R=[cos(theta) sin(theta) 0; -sin(theta) cos(theta) 0; 0 0 1];

e=R*e_w;

== matlab function Switching_02/Unicycle 3/State Feedback Exact Trajectory Controller/Controller/Transformed Inputs ==
  data: SF_b parameter; SF_xi1 parameter; v_d input; w_d input; e input; u1 output; u2 output
function [u1, u2] = fcn(SF_b, SF_xi1, v_d, w_d, e)

% calculatring values of K
k_1=2*SF_xi1*sqrt(SF_b*v_d+w_d^2);
k_2=SF_b;
k_3=k_1;

% calculating values of u
u1=-k_1*e(1);
u2=-k_2*(v_d*(sin(e(3))/e(3)))*e(2)-k_3*e(3);

== matlab function Switching_02/Unicycle 3/State Feedback Exact Trajectory Controller/Differential Flatness/Subsystem1/MATLAB Function ==
  data: u input; u output
function u = fcn(u)

if abs(u)<1e-4
    if u>=0
        u=1e-4;
    else
        u=-1e-4;
    end
else
    u=u;
end

== matlab function Switching_02/Unicycle 2/State Feedback Exact Trajectory Controller/Controller/Inverse Transformation ==
  data: v_d input; w_d input; u1 input; v output size=1; u2 input; w output size=1; e input
function [v, w] = fcn(v_d, w_d, u1, u2, e)

v = v_d*cos(e(3))-u1;
w=w_d-u2;

== matlab function Switching_02/Unicycle 2/State Feedback Exact Trajectory Controller/Controller/MATLAB Function ==
  data: e_w input; e output; theta input
function e  = fcn(e_w, theta)

R=[cos(theta) sin(theta) 0; -sin(theta) cos(theta) 0; 0 0 1];

e=R*e_w;

== matlab function Switching_02/Unicycle 3/State Feedback Exact Trajectory Controller/Controller/Inverse Transformation ==
  data: v_d input; w_d input; u1 input; v output size=1; u2 input; w output size=1; e input
function [v, w] = fcn(v_d, w_d, u1, u2, e)

v = v_d*cos(e(3))-u1;
w=w_d-u2;

== matlab function Switching_02/Swittching Logic ==
  data: switching output; x1 input; x2 input; x3 input; y1 input; y2 input; y3 input; x_d input; y_d input; switching_out input; tolerance_position parameter
function switching = fcn(x1, x2, x3, y1, y2, y3, x_d, y_d, switching_out, tolerance_position)
if switching_out==1
    switching=1;
else
    if sqrt((x1-x_d)^2+(y1-y_d)^2)<tolerance_position && sqrt((x2-x_d)^2+(y2-y_d)^2)<tolerance_position && sqrt((x3-x_d)^2+(y3-y_d)^2)<tolerance_position
        switching = 1; 
    else
        switching = 0; 
    end
end

== matlab function Switching_02/Unicycle 1/State Feedback Exact Trajectory Controller/Controller/Inverse Transformation ==
  data: v_d input; w_d input; u1 input; v output size=1; u2 input; w output size=1; e input
function [v, w] = fcn(v_d, w_d, u1, u2, e)

v = v_d*cos(e(3))-u1;
w=w_d-u2;

== matlab function Switching_02/Unicycle 1/State Feedback Exact Trajectory Controller/Controller/MATLAB Function ==
  data: e_w input; e output; theta input
function e  = fcn(e_w, theta)

R=[cos(theta) sin(theta) 0; -sin(theta) cos(theta) 0; 0 0 1];

e=R*e_w;

== matlab function Switching_02/Unicycle 1/State Feedback Exact Trajectory Controller/Controller/Transformed Inputs ==
  data: SF_b parameter; SF_xi1 parameter; v_d input; w_d input; e input; u1 output; u2 output
function [u1, u2] = fcn(SF_b, SF_xi1, v_d, w_d, e)

% calculatring values of K
k_1=2*SF_xi1*sqrt(SF_b*v_d+w_d^2);
k_2=SF_b;
k_3=k_1;

% calculating values of u
u1=-k_1*e(1);
u2=-k_2*(v_d*(sin(e(3))/e(3)))*e(2)-k_3*e(3);
